simulink model "sw_nl_fcn_anwendung"  (R2020b)
settings: Solver=ode45  StartTime=0.0  StopTime=40.0  MaxStep=0.01  RelTol=1e-3  EnableMultiTasking=on
model workspace (MAT data in the model file):
  k = 1
values from neighbouring files (symbols this model uses):
  A = 2    [sw_nl_fcn_data.m]
  c = 1    [sw_nl_fcn_data.m]
  delta = 0.2    [sw_nl_fcn_data.m]
  w = 3    [sw_nl_fcn_data.m]
settings Model: Creator=Reichl  LastModifiedBy=jakob
settings DataIOCC: LimitDataPoints=on  SaveFormat=Array  SignalLoggingSaveFormat=ModelDataLogs  ReturnWorkspaceOutputs=off
settings OptimizationCC: ExpressionDepthLimit=2147483647  LifeSpan=inf
settings DebuggingCC: UnderspecifiedInitializationDetection=Classic  MergeDetectMultiDrivingBlocksExec=none  SolverPrmCheckMsg=warning  FcnCallInpInsideContextMsg=warning  StateNameClashWarn=warning  SFUnexpectedBacktrackingDiag=warning  SFNoUnconditionalDefaultTransitionDiag=warning  SFExecutionAtInitializationDiag=none  ArithmeticOperatorsInVariantConditions=warning
settings HardwareCC: ProdBitPerPointer=32  ProdBitPerSizeT=32  ProdBitPerPtrDiffT=32  ProdLargestAtomicFloat=None  ProdIntDivRoundTo=Undefined  ProdEndianess=Unspecified  ProdWordSize=32  ProdHWDeviceType=32-bit Generic
settings ModelReferenceCC: PropagateSignalLabelsOutOfModel=off
settings SFSimCC: SimUseLocalCustomCode=off  CustomCodeUndefinedFunction=UseInterfaceOnly
settings RTWCC: RTWUseLocalCustomCode=off
settings CodeAppCC: StateflowObjectComments=on
settings GRTTargetCC: TargetLangStandard=C89/C90 (ANSI)  CombineOutputUpdateFcns=off  GRTInterface=on
settings ConfigComp: CovMetricSettings=dw  CovSaveCumulativeToWorkspaceVar=on  CovSaveSingleToWorkspaceVar=on  CovExternalEMLEnable=off  CovSFcnEnable=off

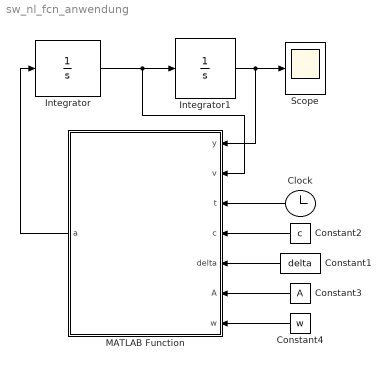
== system sw_nl_fcn_anwendung ==
  Clock : Clock
  Constant1 : Constant  Value=delta
  Constant2 : Constant  Value=c
  Constant3 : Constant  Value=A
  Constant4 : Constant  Value=w
  Integrator : Integrator
  Integrator1 : Integrator  InitialCondition=3
  MATLAB Function : MATLAB Function  TreatAsAtomicUnit=on
  Scope : Scope
  wires:
  Integrator/1 -> MATLAB Function/2(v), Integrator1/1
  Integrator1/1 -> Scope/1, MATLAB Function/1(y)
  MATLAB Function/1(a) -> Integrator/1
  Constant2/1 -> MATLAB Function/4(c)
  Constant4/1 -> MATLAB Function/7(w)
  Constant3/1 -> MATLAB Function/6(A)
  Constant1/1 -> MATLAB Function/5(delta)
  Clock/1 -> MATLAB Function/3(t)

== matlab function sw_nl_fcn_anwendung/MATLAB Function ==
  data: y input; v input; t input; a output; c input; delta input; A input; w input
function a = fcn(y,v,t,c,delta,A,w)
% berechne die Beschleunigung
a = -2*delta*v-c*y+A*sin(w*t)
